simulink model "Schema_a_blocchi_tesina"  (R2023b)
settings: Solver=VariableStepAuto  StartTime=0.0  StopTime=1000  RelTol=1e-3
values from neighbouring files (symbols this model uses):
  C1 = 5    [Modello_idraulico.m]    (also in ciccio_ciccio.m = 0.1; tesina.m = 50)
  C2 = 10    [Modello_idraulico.m]    (also in ciccio_ciccio.m = 1; tesina.m = 25)
  R12 = 5    [tesina.m]
  R1e = 10    [tesina.m]
  R1i = 1    [tesina.m]
  R2e = 12    [tesina.m]
  R2i = 1    [tesina.m]
settings Model: Creator=simon  LastModifiedBy=simon

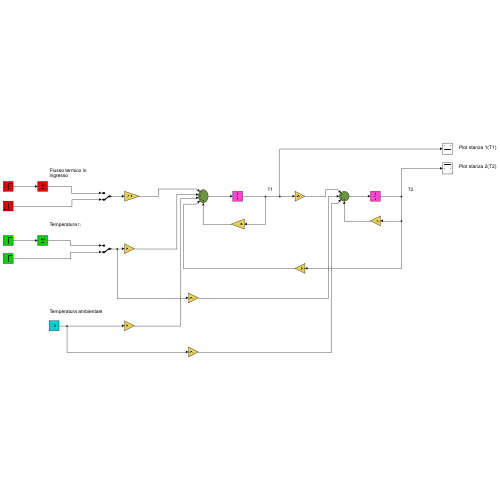
[thumbnail: Simulink's stored preview of the top-level diagram]
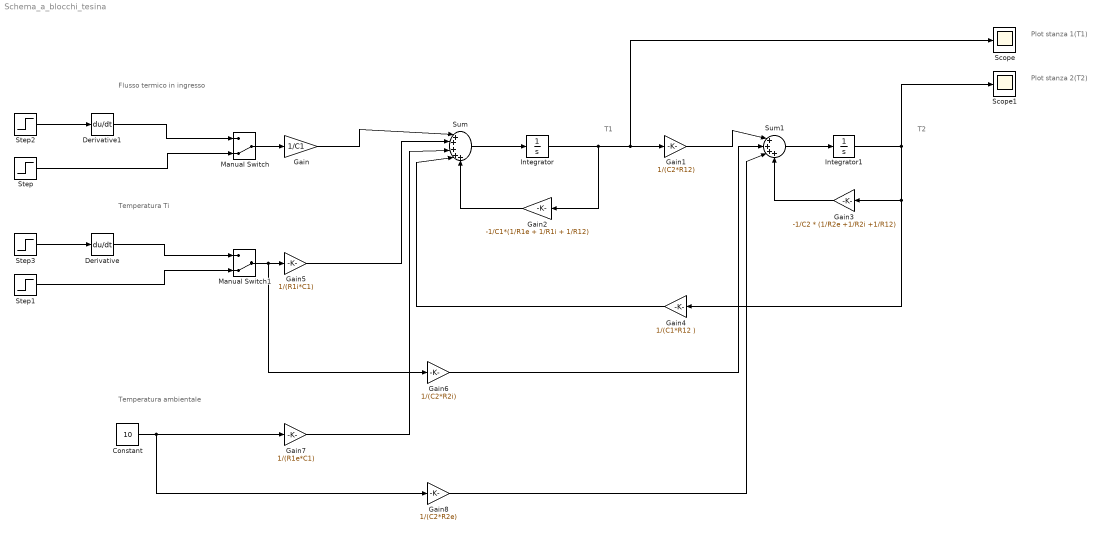
== system Schema_a_blocchi_tesina ==
  note: T2
  note: T1
  note: Plot stanza 2(T2)
  note: Plot stanza 1(T1)
  note: Temperatura ambientale
  note: Temperatura Ti
  note: Flusso termico in ingresso
  Constant : Constant  Value=10
  Derivative : Derivative
  Derivative1 : Derivative
  Gain : Gain  Gain=1/C1
  Gain1 : Gain  Gain=1/(C2*R12)
  Gain2 : Gain  Gain=-1/C1*(1/R1e + 1/R1i + 1/R12)
  Gain3 : Gain  Gain=-1/C2 * (1/R2e +1/R2i +1/R12)
  Gain4 : Gain  Gain=1/(C1*R12 )
  Gain5 : Gain  Gain=1/(R1i*C1)
  Gain6 : Gain  Gain=1/(C2*R2i)
  Gain7 : Gain  Gain=1/(R1e*C1)
  Gain8 : Gain  Gain=1/(C2*R2e)
  Integrator : Integrator
  Integrator1 : Integrator
  Manual Switch : ManualSwitch  CurrentSetting=0
  Manual Switch1 : ManualSwitch  CurrentSetting=0
  Scope : Scope
  Scope1 : Scope
  Step : Step  Time=10  After=10  SampleTime=0
  Step1 : Step  Time=10  After=15  SampleTime=0
  Step2 : Step  SampleTime=0
  Step3 : Step  SampleTime=0
  Sum : Sum  Inputs=|+++++
  Sum1 : Sum  Inputs=|++++
  wires:
  Derivative1/1 -> Manual Switch/1
  Step/1 -> Manual Switch/2
  Manual Switch/1 -> Gain/1
  Gain/1 -> Sum/1
  Sum/1 -> Integrator/1
  Integrator/1 -> Scope/1, Gain1/1, Gain2/1
  Gain2/1 -> Sum/5
  Gain1/1 -> Sum1/1
  Sum1/1 -> Integrator1/1
  Gain3/1 -> Sum1/4
  Integrator1/1 -> Scope1/1, Gain4/1, Gain3/1
  Gain4/1 -> Sum/4
  Step1/1 -> Manual Switch1/2
  Derivative/1 -> Manual Switch1/1
  Gain5/1 -> Sum/2
  Manual Switch1/1 -> Gain6/1, Gain5/1
  Gain6/1 -> Sum1/2
  Constant/1 -> Gain8/1, Gain7/1
  Gain7/1 -> Sum/3
  Gain8/1 -> Sum1/3
  Step2/1 -> Derivative1/1
  Step3/1 -> Derivative/1
